simulink model "GVCU_HIL"  (R2026a)
settings: Solver=ode3  StartTime=0  StopTime=2474  FixedStep=0.0002
model workspace (MAT data in the model file):
  CANoelibParameters : object (value not decoded)
values from neighbouring files (symbols this model uses):
  acc_pedal_data = pedal_data.accelerator_pedal_position_t0    [Vehicle_Simulink_init.m]
  acc_pedal_time = pedal_data.t0    [Vehicle_Simulink_init.m]
  brk_pedal_data = brake_pedal_data.shared_brakes_drvrBrkPedlPerc_t0    [Vehicle_Simulink_init.m]
  brk_pedal_time = brake_pedal_data.t0    [Vehicle_Simulink_init.m]
  cycle_len = zeros(1, num_cycles)    [Vehicle_Simulink_init.m]
  cycle_speed_matrix = zeros(max_cycle_len, num_cycles)    [Vehicle_Simulink_init.m]
  cycle_time_matrix = zeros(max_cycle_len, num_cycles)    [Vehicle_Simulink_init.m]
  veh_speed_data = speed_data.shared_dynamicsVso_vehVelLgt_t0    [Vehicle_Simulink_init.m]
  veh_speed_time = speed_data.t0    [Vehicle_Simulink_init.m]
undefined symbols (not defined in the file or in its folder): Active, AuxActive, bat, environment, FL_prs_voltage, FR_prs_voltage, pos, RL_prs_voltage, RR_prs_voltage, tir, veh, VGetRawValueFlag, Voltage, VT2816_1_Ch1, VT2816_1_Ch2, VT2816_1_Ch3, VT2816_1_Ch4, VT2816_3_Ch13, VT2816_3_Ch14, VT7101_1_Out2, VT7820_2_Channel1, VT7820_2_Channel2, VT7820_2_Channel3, VT7820_2_Channel4, VTS
libraries: canoelib x144, autolibsharedcoupling x21, autolibcoupling x9, autolibshared x5, simulink_extras x4, simulink x4, slpidlib x3, autolibshareddiff x3, autolibutils x1, autolibdatasheetbattery x1, autolibmappedmotor x1, sl_discontinuities x1
(part 2 of 9)

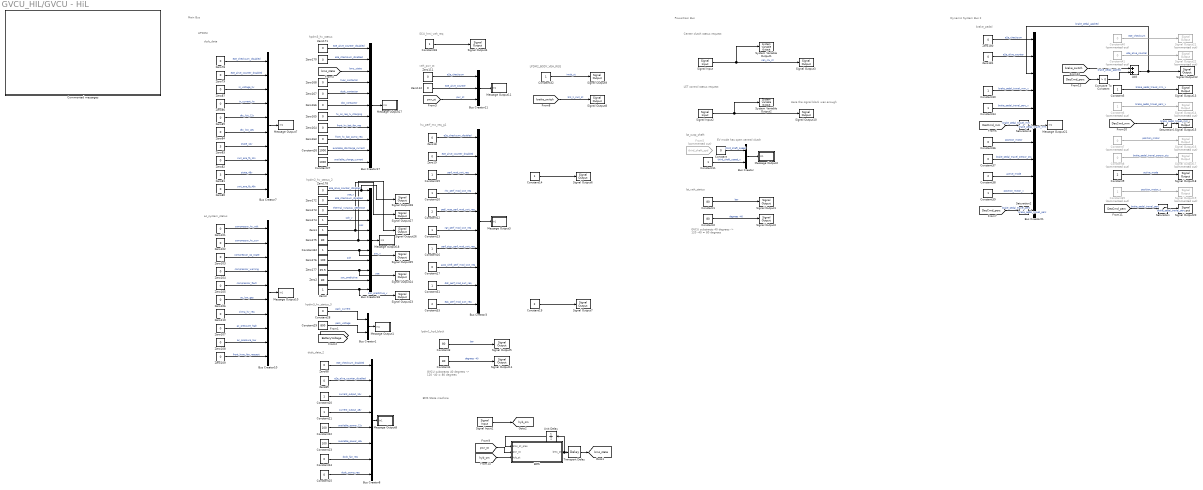
== system GVCU_HIL/GVCU - HiL ==
  note: EV mode has open central clutch
  note: GVCU substracts 40 degrees
      | -> 120 -40 =  80 degrees
  note: hu_perf_mo_req_g1
  note: HPDM3
  note: hpdm2_hv_status_2
  note: dcdc_data
  note: hpdm3_hv_status_3
  note: dcdc_data_2
  note: Here the signal block was enough
  note: ac_system_status
  note: LPDM2_BODY_VEH_REQ
  note: brake_pedal
  note: veh_pwr_st
  note: hpdm3_hv_status
  note: lst_outp_shaft
  note: Powertrain Bus
  note: Center clutch status request
  note: SCU_hmi_veh_req
  note: LST control status request
  note: Main Bus
  note: Dynamic System Bus 2
  note: lst_veh_status
  note: lpdm1_hyd_block
  note: GVCU substracts 40 degrees
      | -> 120 -40 =  80 degrees
  note: BMS State machine
  Add : Sum
  BMS : MATLAB Function  TreatAsAtomicUnit=on
  Bus Creator : BusCreator  Inputs=2
  Bus Creator1 : BusCreator  Inputs=2
  Bus Creator10 : BusCreator  Inputs=10
  Bus Creator11 : BusCreator  Inputs=3
  Bus Creator17 : BusCreator  Inputs=11
  Bus Creator18 : BusCreator  Inputs=11
  Bus Creator21 : BusCreator  Inputs=11
  Bus Creator3 : BusCreator  Inputs=10
  Bus Creator7 : BusCreator  Inputs=10
  Bus Creator8 : BusCreator  Inputs=8
  Commented messages : Subsystem
  Compare To Constant : simulink/Logic and Bit Operations/Compare To Constant  relop=>  const=0  OutDataTypeStr=boolean
  Constant{,17,24..25,28,36..37} (7 alike) : Constant  Value=0
  Constant{1..4} (4 alike) : Constant  Value=80
  Constant{5,10..11,13..16,18,20..21,30..32,34,39,42} (16 alike) : Constant
  Constant{9,12,19,33,38} (5 alike) : Constant  Value=2
  Constant22 : Constant  Value=100
  Constant23 : Constant  Value=100
  Constant26 : Constant  Value=1000
  Constant27 : Constant  Value=1000
  Constant29 : Constant  Value=800
  Constant35 : Constant  Commented=on
  Constant{7..8,40..41} (4 alike) : Constant  Commented=on  Value=0
  Constant6 : Constant  Commented=on
  From5 : From  Commented=on  GotoTag=third_shaft_spd
  Message Output1 : Subsystem  AncestorBlock=canoelib/CANoe I//O/Message Output  mask(Signal Output Module){dbName=main_bus, nodeName=HPDM3, msgName=hpdm3_hv_status_3, inputType=Bus Signal, rawValue=Default}
      mask prompts: dbName "Database name"; nodeName "Node name"; msgName "Message name"; inputType "Input type"; rawValue "Raw value"
      mask help: Output module for all signals of a databasemessage provided by the CANoe interaction layer. Double click the block for configuration.
      settings: AttributesFormatString=%<msgName>  CopyFcn=set_param(gcb, 'AttributesFormatString', '%<msgName>');  OpenFcn=MessageOutputBlock
      mask Help: For detailed information please refer to the CANoe online help 'MATLAB Integration Package » CANoe I/O Library'.
      mask TypeOptions inputType: Vector | Bus Signal
      mask TypeOptions rawValue: Default | Physical value | Raw value
      mask Display:
      | image(imread('MatlabBlock.png'))
      | disp('CANoe')
  Message Output10 : Subsystem  AncestorBlock=canoelib/CANoe I//O/Message Output  mask(Signal Output Module){dbName=main_bus, nodeName=LPDM1, msgName=ac_system_status, inputType=Bus Signal, rawValue=Default}
      mask prompts: dbName "Database name"; nodeName "Node name"; msgName "Message name"; inputType "Input type"; rawValue "Raw value"
      mask help: Output module for all signals of a databasemessage provided by the CANoe interaction layer. Double click the block for configuration.
      settings: AttributesFormatString=%<msgName>  CopyFcn=set_param(gcb, 'AttributesFormatString', '%<msgName>');  OpenFcn=MessageOutputBlock
      mask Help: For detailed information please refer to the CANoe online help 'MATLAB Integration Package » CANoe I/O Library'.
      mask TypeOptions inputType: Vector | Bus Signal
      mask TypeOptions rawValue: Default | Physical value | Raw value
      mask Display:
      | image(imread('MatlabBlock.png'))
      | disp('CANoe')
  Message Output11 : Subsystem  AncestorBlock=canoelib/CANoe I//O/Message Output  mask(Signal Output Module){dbName=main_bus, nodeName=SCU, msgName=veh_pwr_st, inputType=Bus Signal, rawValue=Default}
      mask prompts: dbName "Database name"; nodeName "Node name"; msgName "Message name"; inputType "Input type"; rawValue "Raw value"
      mask help: Output module for all signals of a databasemessage provided by the CANoe interaction layer. Double click the block for configuration.
      settings: AttributesFormatString=veh_pwr_st  CopyFcn=set_param(gcb, 'AttributesFormatString', '%<msgName>');  OpenFcn=MessageOutputBlock
      mask Help: For detailed information please refer to the CANoe online help 'MATLAB Integration Package » CANoe I/O Library'.
      mask TypeOptions inputType: Vector | Bus Signal
      mask TypeOptions rawValue: Default | Physical value | Raw value
      mask Display:
      | image(imread('MatlabBlock.png'))
      | disp('CANoe')
  Message Output17 : Subsystem  AncestorBlock=canoelib/CANoe I//O/Message Output  mask(Signal Output Module){dbName=main_bus, nodeName=HPDM3, msgName=hpdm3_hv_status, inputType=Bus Signal, rawValue=Default}
      mask prompts: dbName "Database name"; nodeName "Node name"; msgName "Message name"; inputType "Input type"; rawValue "Raw value"
      mask help: Output module for all signals of a databasemessage provided by the CANoe interaction layer. Double click the block for configuration.
      settings: AttributesFormatString=%<msgName>  CopyFcn=set_param(gcb, 'AttributesFormatString', '%<msgName>');  OpenFcn=MessageOutputBlock
      mask Help: For detailed information please refer to the CANoe online help 'MATLAB Integration Package » CANoe I/O Library'.
      mask TypeOptions inputType: Vector | Bus Signal
      mask TypeOptions rawValue: Default | Physical value | Raw value
      mask Display:
      | image(imread('MatlabBlock.png'))
      | disp('CANoe')
  Message Output18 : Subsystem  AncestorBlock=canoelib/CANoe I//O/Message Output  mask(Signal Output Module){dbName=main_bus, nodeName=HPDM3, msgName=hpdm3_hv_status_2, inputType=Bus Signal, rawValue=Default}
      mask prompts: dbName "Database name"; nodeName "Node name"; msgName "Message name"; inputType "Input type"; rawValue "Raw value"
      mask help: Output module for all signals of a databasemessage provided by the CANoe interaction layer. Double click the block for configuration.
      settings: AttributesFormatString=hpdm3_hv_status_2  CopyFcn=set_param(gcb, 'AttributesFormatString', '%<msgName>');  OpenFcn=MessageOutputBlock
      mask Help: For detailed information please refer to the CANoe online help 'MATLAB Integration Package » CANoe I/O Library'.
      mask TypeOptions inputType: Vector | Bus Signal
      mask TypeOptions rawValue: Default | Physical value | Raw value
      mask Display:
      | image(imread('MatlabBlock.png'))
      | disp('CANoe')
  Message Output2 : Subsystem  AncestorBlock=canoelib/CANoe I//O/Message Output  mask(Signal Output Module){dbName=powertrain_bus, nodeName=LST, msgName=lst_outp_shaft, inputType=Bus Signal, rawValue=Default}
      mask prompts: dbName "Database name"; nodeName "Node name"; msgName "Message name"; inputType "Input type"; rawValue "Raw value"
      mask help: Output module for all signals of a databasemessage provided by the CANoe interaction layer. Double click the block for configuration.
      settings: AttributesFormatString=%<msgName>  CopyFcn=set_param(gcb, 'AttributesFormatString', '%<msgName>');  OpenFcn=MessageOutputBlock
      mask Help: For detailed information please refer to the CANoe online help 'MATLAB Integration Package » CANoe I/O Library'.
      mask TypeOptions inputType: Vector | Bus Signal
      mask TypeOptions rawValue: Default | Physical value | Raw value
      mask Display:
      | image(imread('MatlabBlock.png'))
      | disp('CANoe')
  Message Output21 : Subsystem  AncestorBlock=canoelib/CANoe I//O/Message Output  mask(Signal Output Module){dbName=dynamic_systems2_bus, nodeName=IEB, msgName=brake_pedal, inputType=Bus Signal, rawValue=Default}
      mask prompts: dbName "Database name"; nodeName "Node name"; msgName "Message name"; inputType "Input type"; rawValue "Raw value"
      mask help: Output module for all signals of a databasemessage provided by the CANoe interaction layer. Double click the block for configuration.
      settings: AttributesFormatString=brake_pedal  CopyFcn=set_param(gcb, 'AttributesFormatString', '%<msgName>');  OpenFcn=MessageOutputBlock
      mask Help: For detailed information please refer to the CANoe online help 'MATLAB Integration Package » CANoe I/O Library'.
      mask TypeOptions inputType: Vector | Bus Signal
      mask TypeOptions rawValue: Default | Physical value | Raw value
      mask Display:
      | image(imread('MatlabBlock.png'))
      | disp('CANoe')
  Message Output3 : Subsystem  AncestorBlock=canoelib/CANoe I//O/Message Output  mask(Signal Output Module){dbName=main_bus, nodeName=SCU, msgName=hu_perf_mod_req_g1, inputType=Bus Signal, rawValue=Default}
      mask prompts: dbName "Database name"; nodeName "Node name"; msgName "Message name"; inputType "Input type"; rawValue "Raw value"
      mask help: Output module for all signals of a databasemessage provided by the CANoe interaction layer. Double click the block for configuration.
      settings: AttributesFormatString=%<msgName>  CopyFcn=set_param(gcb, 'AttributesFormatString', '%<msgName>');  OpenFcn=MessageOutputBlock
      mask Help: For detailed information please refer to the CANoe online help 'MATLAB Integration Package » CANoe I/O Library'.
      mask TypeOptions inputType: Vector | Bus Signal
      mask TypeOptions rawValue: Default | Physical value | Raw value
      mask Display:
      | image(imread('MatlabBlock.png'))
      | disp('CANoe')
  Message Output7 : Subsystem  AncestorBlock=canoelib/CANoe I//O/Message Output  mask(Signal Output Module){dbName=main_bus, nodeName=HPDM3, msgName=dcdc_data, inputType=Bus Signal, rawValue=Default}
      mask prompts: dbName "Database name"; nodeName "Node name"; msgName "Message name"; inputType "Input type"; rawValue "Raw value"
      mask help: Output module for all signals of a databasemessage provided by the CANoe interaction layer. Double click the block for configuration.
      settings: AttributesFormatString=%<msgName>  CopyFcn=set_param(gcb, 'AttributesFormatString', '%<msgName>');  OpenFcn=MessageOutputBlock
      mask Help: For detailed information please refer to the CANoe online help 'MATLAB Integration Package » CANoe I/O Library'.
      mask TypeOptions inputType: Vector | Bus Signal
      mask TypeOptions rawValue: Default | Physical value | Raw value
      mask Display:
      | image(imread('MatlabBlock.png'))
      | disp('CANoe')
  Message Output8 : Subsystem  AncestorBlock=canoelib/CANoe I//O/Message Output  mask(Signal Output Module){dbName=main_bus, nodeName=HPDM3, msgName=dcdc_data_2, inputType=Bus Signal, rawValue=Default}
      mask prompts: dbName "Database name"; nodeName "Node name"; msgName "Message name"; inputType "Input type"; rawValue "Raw value"
      mask help: Output module for all signals of a databasemessage provided by the CANoe interaction layer. Double click the block for configuration.
      settings: AttributesFormatString=%<msgName>  CopyFcn=set_param(gcb, 'AttributesFormatString', '%<msgName>');  OpenFcn=MessageOutputBlock
      mask Help: For detailed information please refer to the CANoe online help 'MATLAB Integration Package » CANoe I/O Library'.
      mask TypeOptions inputType: Vector | Bus Signal
      mask TypeOptions rawValue: Default | Physical value | Raw value
      mask Display:
      | image(imread('MatlabBlock.png'))
      | disp('CANoe')
  Saturation : Saturate  UpperLimit=100  LowerLimit=0
  Saturation1 : Saturate  UpperLimit=25.5  LowerLimit=0
  Saturation2 : Saturate  UpperLimit=100  LowerLimit=0
  Saturation3 : Saturate  UpperLimit=25.5  LowerLimit=0
  Signal Input : canoelib/CANoe I//O/Signal Input  dbName=powertrain_bus  nodeName=GVCU  msgName=gvcu_lst_req  sigName=cen_clu_st_req  editSampleTime=0  rawValue=Default  dataType=Default  dataTypeDB=uint8  hasEncoding=off
      settings: AttributesFormatString=%<sigName>  SourceProductName=Vector CANoe
  Signal Input1 : canoelib/CANoe I//O/Signal Input  dbName=main_bus  nodeName=GVCU  msgName=gvcu_hv_control  sigName=hyb_st_mac_state  editSampleTime=0  rawValue=Default  dataType=Default  dataTypeDB=uint8  hasEncoding=off
      settings: AttributesFormatString=%<sigName>  SourceProductName=Vector CANoe
  Signal Input2 : canoelib/CANoe I//O/Signal Input  dbName=powertrain_bus  nodeName=GVCU  msgName=gvcu_lst_req  sigName=lst_ctrl_st_req  editSampleTime=0  rawValue=Default  dataType=Default  dataTypeDB=uint8  hasEncoding=off
      settings: AttributesFormatString=%<sigName>  SourceProductName=Vector CANoe
  Signal Output1 : canoelib/CANoe I//O/Signal Output  dbName=powertrain_bus  nodeName=LST  msgName=lst_veh_status  sigName=re_hi_p_sys_p  rawValue=Default  dataType=Default  dataTypeDB=uint8  hasEncoding=off
      settings: AttributesFormatString=%<sigName>  SourceProductName=Vector CANoe
  Signal Output10 : canoelib/CANoe I//O/Signal Output  dbName=powertrain_bus  nodeName=LST  msgName=lst_tq_sts_1  sigName=lst_ctrl_st  rawValue=Default  dataType=Default  dataTypeDB=uint8  hasEncoding=off
      settings: AttributesFormatString=%<sigName>  SourceProductName=Vector CANoe
  Signal Output11 : canoelib/CANoe I//O/Signal Output  dbName=main_bus  nodeName=LPDM1  msgName=lpdm1_hyd_block  sigName=autoskin_oil_temperature  rawValue=Default  dataType=Default  dataTypeDB=uint8  hasEncoding=on
      settings: AttributesFormatString=%<sigName>  SourceProductName=Vector CANoe
  Signal Output12 : canoelib/CANoe I//O/Signal Output  dbName=dynamic_systems2_bus  nodeName=IEB  msgName=brake_pedal  sigName=brake_pedal_applied  rawValue=Default  dataType=Default  dataTypeDB=uint8  hasEncoding=off
      settings: AttributesFormatString=%<sigName>  SourceProductName=Vector CANoe
  Signal Output13 : canoelib/CANoe I//O/Signal Output  dbName=dynamic_systems2_bus  nodeName=IEB  msgName=brake_pedal  sigName=brake_pedal_travel_mm_v  rawValue=Default  dataType=Default  dataTypeDB=boolean  hasEncoding=off
      settings: AttributesFormatString=%<sigName>  SourceProductName=Vector CANoe
  Signal Output14 : canoelib/CANoe I//O/Signal Output  Commented=on  dbName=dynamic_systems2_bus  nodeName=IEB  msgName=brake_pedal  sigName=brake_pedal_travel_perc_v  rawValue=Default  dataType=Default  dataTypeDB=boolean  hasEncoding=off
      settings: AttributesFormatString=%<sigName>  SourceProductName=Vector CANoe
  Signal Output15 : canoelib/CANoe I//O/Signal Output  dbName=dynamic_systems2_bus  nodeName=IEB  msgName=brake_pedal  sigName=brake_pedal_travel_mm  rawValue=Default  dataType=Default  dataTypeDB=uint8  hasEncoding=on
      settings: AttributesFormatString=%<sigName>  SourceProductName=Vector CANoe
  Signal Output16 : canoelib/CANoe I//O/Signal Output  Commented=on  dbName=dynamic_systems2_bus  nodeName=IEB  msgName=brake_pedal  sigName=brake_pedal_travel_perc_v  rawValue=Default  dataType=Default  dataTypeDB=boolean  hasEncoding=off
      settings: AttributesFormatString=%<sigName>  SourceProductName=Vector CANoe
  Signal Output17 : canoelib/CANoe I//O/Signal Output  Commented=on  dbName=dynamic_systems2_bus  nodeName=IEB  msgName=brake_pedal  sigName=brake_pedal_travel_sensor_sts  rawValue=Default  dataType=Default  dataTypeDB=uint8  hasEncoding=off
      settings: AttributesFormatString=%<sigName>  SourceProductName=Vector CANoe
  Signal Output18 : canoelib/CANoe I//O/Signal Output  dbName=dynamic_systems2_bus  nodeName=IEB  msgName=brake_pedal  sigName=active_mode  rawValue=Default  dataType=Default  dataTypeDB=uint8  hasEncoding=off
      settings: AttributesFormatString=%<sigName>  SourceProductName=Vector CANoe
  Signal Output19 : canoelib/CANoe I//O/Signal Output  Commented=on  dbName=dynamic_systems2_bus  nodeName=IEB  msgName=brake_pedal  sigName=position_motor_v  rawValue=Default  dataType=Default  dataTypeDB=boolean  hasEncoding=off
      settings: AttributesFormatString=%<sigName>  SourceProductName=Vector CANoe
  Signal Output2 : canoelib/CANoe I//O/Signal Output  dbName=powertrain_bus  nodeName=LST  msgName=lst_veh_status  sigName=re_hi_p_sys_t  rawValue=Default  dataType=Default  dataTypeDB=uint8  hasEncoding=on
      settings: AttributesFormatString=%<sigName>  SourceProductName=Vector CANoe
  Signal Output20 : canoelib/CANoe I//O/Signal Output  dbName=dynamic_systems2_bus  nodeName=IEB  msgName=brake_pedal  sigName=brake_pedal_travel_perc  rawValue=Default  dataType=Default  dataTypeDB=uint16  hasEncoding=on
      settings: AttributesFormatString=%<sigName>  SourceProductName=Vector CANoe
  Signal Output21 : canoelib/CANoe I//O/Signal Output  Commented=on  dbName=dynamic_systems2_bus  nodeName=IEB  msgName=brake_pedal  sigName=e2e_checksum  rawValue=Default  dataType=Default  dataTypeDB=uint8  hasEncoding=off
      settings: AttributesFormatString=%<sigName>  SourceProductName=Vector CANoe
  Signal Output22 : canoelib/CANoe I//O/Signal Output  Commented=on  dbName=dynamic_systems2_bus  nodeName=IEB  msgName=brake_pedal  sigName=e2e_alive_counter  rawValue=Default  dataType=Default  dataTypeDB=uint8  hasEncoding=off
      settings: AttributesFormatString=%<sigName>  SourceProductName=Vector CANoe
  Signal Output23 : canoelib/CANoe I//O/Signal Output  dbName=main_bus  nodeName=HPDM3  msgName=hpdm3_hv_status_2  sigName=soc_predictive_v  rawValue=Default  dataType=Default  dataTypeDB=boolean  hasEncoding=off
      settings: AttributesFormatString=%<sigName>  SourceProductName=Vector CANoe
  Signal Output24 : canoelib/CANoe I//O/Signal Output  dbName=main_bus  nodeName=HPDM3  msgName=hpdm3_hv_status_2  sigName=soe  rawValue=Default  dataType=Default  dataTypeDB=uint8  hasEncoding=on
      settings: AttributesFormatString=%<sigName>  SourceProductName=Vector CANoe
  Signal Output25 : canoelib/CANoe I//O/Signal Output  dbName=main_bus  nodeName=HPDM3  msgName=hpdm3_hv_status_2  sigName=soc_v  rawValue=Default  dataType=Default  dataTypeDB=boolean  hasEncoding=off
      settings: AttributesFormatString=%<sigName>  SourceProductName=Vector CANoe
  Signal Output26 : canoelib/CANoe I//O/Signal Output  dbName=main_bus  nodeName=HPDM3  msgName=hpdm3_hv_status_2  sigName=soc  rawValue=Default  dataType=Default  dataTypeDB=uint16  hasEncoding=on
      settings: AttributesFormatString=%<sigName>  SourceProductName=Vector CANoe
  Signal Output27 : canoelib/CANoe I//O/Signal Output  dbName=main_bus  nodeName=HPDM3  msgName=hpdm3_hv_status_2  sigName=soe_v  rawValue=Default  dataType=Default  dataTypeDB=boolean  hasEncoding=off
      settings: AttributesFormatString=%<sigName>  SourceProductName=Vector CANoe
  Signal Output28 : canoelib/CANoe I//O/Signal Output  dbName=main_bus  nodeName=HPDM3  msgName=hpdm3_hv_status_2  sigName=e2e_alive_counter_disabled  rawValue=Default  dataType=Default  dataTypeDB=uint8  hasEncoding=off
      settings: AttributesFormatString=%<sigName>  SourceProductName=Vector CANoe
  Signal Output3 : canoelib/CANoe I//O/Signal Output  dbName=powertrain_bus  nodeName=LST  msgName=lst_tq_sts_2  sigName=cen_clu_st  rawValue=Default  dataType=Default  dataTypeDB=uint8  hasEncoding=off
      settings: AttributesFormatString=%<sigName>  SourceProductName=Vector CANoe
  Signal Output4 : canoelib/CANoe I//O/Signal Output  dbName=main_bus  nodeName=SCU  msgName=scu_hmi_veh_req  sigName=suppg_mod_req  rawValue=Default  dataType=Default  dataTypeDB=uint8  hasEncoding=off
      settings: AttributesFormatString=%<sigName>  SourceProductName=Vector CANoe
  Signal Output5 : canoelib/CANoe I//O/Signal Output  dbName=main_bus  nodeName=LPDM1  msgName=lpdm1_hyd_block  sigName=autoskin_oil_pressure  rawValue=Default  dataType=Default  dataTypeDB=uint16  hasEncoding=on
      settings: AttributesFormatString=%<sigName>  SourceProductName=Vector CANoe
  Signal Output6 : canoelib/CANoe I//O/Signal Output  dbName=main_bus  nodeName=SCU  msgName=hu_perf_mod_req_g1  sigName=perf_mod_swt_req  rawValue=Default  dataType=Default  dataTypeDB=uint8  hasEncoding=off
      settings: AttributesFormatString=%<sigName>  SourceProductName=Vector CANoe
  Signal Output7 : canoelib/CANoe I//O/Signal Output  dbName=main_bus  nodeName=SCU  msgName=hu_perf_mod_req_g1  sigName=eps_perf_mod_swt_req  rawValue=Default  dataType=Default  dataTypeDB=uint8  hasEncoding=off
      settings: AttributesFormatString=%<sigName>  SourceProductName=Vector CANoe
  Signal Output8 : canoelib/CANoe I//O/Signal Output  dbName=main_bus  nodeName=LPDM2  msgName=lpdm2_body_veh_req  sigName=brk_li_swt_st  rawValue=Default  dataType=Default  dataTypeDB=uint8  hasEncoding=off
      settings: AttributesFormatString=%<sigName>  SourceProductName=Vector CANoe
  Signal Output9 : canoelib/CANoe I//O/Signal Output  dbName=main_bus  nodeName=LPDM2  msgName=lpdm2_body_veh_req  sigName=imob_st  rawValue=Default  dataType=Default  dataTypeDB=uint8  hasEncoding=off
      settings: AttributesFormatString=%<sigName>  SourceProductName=Vector CANoe
  System Variable Output1 : canoelib/CANoe I//O/System Variable Output  nsName=Checker_Simulink  sysVarName=cen_clu_st  arrayIndex=-1  rawValue=Default  dataType=Default  dataTypeDB=int32  hasEncoding=off  dataTypeCANoe=Get from CANoe
      settings: AttributesFormatString=%<nsName>::%<sysVarName>  SourceProductName=Vector CANoe
  System Variable Output2 : canoelib/CANoe I//O/System Variable Output  nsName=Checker_Simulink  sysVarName=lst_ctrl_st  arrayIndex=-1  rawValue=Default  dataType=Default  dataTypeDB=int32  hasEncoding=off  dataTypeCANoe=Get from CANoe
      settings: AttributesFormatString=%<nsName>::%<sysVarName>  SourceProductName=Vector CANoe
  Transport Delay : TransportDelay
  Unit Delay : UnitDelay  SampleTime=-1
  Zero1 : Constant  OutDataTypeStr=Inherit: Inherit via back propagation
  Zero{18..19,78..80,82,84..89,101..112,163..168,170..173,178,180..181} (37 alike) : Constant  Value=0  OutDataTypeStr=Inherit: Inherit via back propagation
  Zero174 : Constant  OutDataTypeStr=Inherit: Inherit via back propagation
  Zero175 : Constant  Value=80  OutDataTypeStr=Inherit: Inherit via back propagation
  Zero176 : Constant  Value=100  OutDataTypeStr=Inherit: Inherit via back propagation
  Zero177 : Constant  Value=25.5  OutDataTypeStr=Inherit: Inherit via back propagation
  Zero2 : Constant  Value=80  OutDataTypeStr=Inherit: Inherit via back propagation
  Zero3 : Constant  OutDataTypeStr=Inherit: Inherit via back propagation
  Zero81 : Constant  Value=3  OutDataTypeStr=Inherit: Inherit via back propagation
  Zero83 : Constant  Value=3  OutDataTypeStr=Inherit: Inherit via back propagation
  tag scope: bms_state=global, hyb_sm=global
  wires:
  Zero165/1 -> Bus Creator17/7  "hv_on_req_lv_charging"
  Zero104/1 -> Bus Creator10/4  "compressor_warning"
  Constant38/1 -> Bus Creator21/9  "active_mode"
  Zero103/1 -> Bus Creator10/3  "compressor_op_state"
  Zero109/1 -> Bus Creator10/10  "front_hvac_fan_request"
  Constant34/1 -> Bus Creator21/5  "brake_pedal_travel_perc_v"
  Constant33/1 -> Bus Creator3/10  "eps_perf_mod_swt_req"
  Zero79/1 -> Bus Creator7/2  "e2e_alive_counter_disabled"
  Constant30/1 -> Bus Creator21/4  "brake_pedal_travel_mm_v"
  Zero173/1 -> Bus Creator18/3  "thermal_runaway_detection"
  Constant16/1 -> Bus Creator3/7  "perf_stgy_perf_mod_swt_req"
  Zero180/1 -> Bus Creator21/1  "e2e_checksum"
  [bms_state] -> Bus Creator17/3  "bms_state"
  Zero164/1 -> Bus Creator17/8  "front_hv_bat_fan_req"
  Constant22/1 -> Bus Creator8/5  "available_power_12v"
  Constant36/1 -> Bus Creator21/7  "position_motor"
  Constant24/1 -> Bus Creator8/7  "dcdc_fan_req"
  Constant31/1 -> Bus Creator3/9  "ddc_perf_mod_swt_req"
  Constant39/1 -> Bus Creator21/10  "position_motor_v"
  Constant15/1 -> Bus Creator3/3  "perf_mod_swt_req"
  Bus Creator18/1 -> Message Output18/1(In1)
  Zero111/1 -> Bus Creator11/1  "e2e_checksum"
  Zero86/1 -> Bus Creator7/4  "in_current_hv"
  Constant37/1 -> Bus Creator21/8  "brake_pedal_travel_sensor_sts"
  Zero81/1 -> Bus Creator7/9  "state_48v"
  Zero83/1 -> Bus Creator7/7  "state_12v"
  Constant21/1 -> Bus Creator8/4  "current_output_48v"
  Zero177/1 -> Signal Output24/1, Bus Creator18/9  "soe"
  Zero89/1 -> Bus Creator8/2  "e2e_alive_counter_disabled"
  Signal Input/1 -> Signal Output3/1, System Variable Output1/1  "cen_clu_st"
  Zero88/1 -> Bus Creator8/1  "e2e_checksum_disabled"
  Constant14/1 -> Signal Output6/1
  Bus Creator3/1 -> Message Output3/1(In1)
  Zero176/1 -> Bus Creator18/8  "soh"
  Zero80/1 -> Bus Creator7/10  "swt_ena_fb_48v"
  Zero178/1 -> Signal Output28/1, Bus Creator18/1  "e2e_alive_counter_disabled"
  Zero101/1 -> Bus Creator10/1  "compressor_hv_volt"
  Zero168/1 -> Bus Creator17/4  "hvac_contactor"
  Zero175/1 -> Signal Output26/1, Bus Creator18/6  "soc"
  Bus Creator1/1 -> Message Output1/1(In1)
  Add/1 -> Bus Creator21/3, Signal Output12/1  "brake_pedal_applied"
  Zero18/1 -> Bus Creator3/1  "e2e_checksum_disabled"
  Constant19/1 -> Signal Output7/1
  Zero181/1 -> Bus Creator21/2  "e2e_alive_counter"
  Zero105/1 -> Bus Creator10/5  "compressor_fault"
  Bus Creator7/1 -> Message Output7/1(In1)
  Zero87/1 -> Bus Creator7/3  "in_voltage_hv"
  Constant18/1 -> Signal Output4/1
  Zero82/1 -> Bus Creator7/8  "swt_ena_fb_12v"
  Zero163/1 -> Bus Creator17/9  "front_hv_bat_pump_req"
  Constant27/1 -> Bus Creator17/11  "available_charge_current"
  Zero19/1 -> Bus Creator3/2  "e2e_alive_counter_disabled"
  Bus Creator10/1 -> Message Output10/1(In1)
  Constant26/1 -> Bus Creator17/10  "available_discharge_current"
  Zero174/1 -> Bus Creator18/4  "soh_v"
  Bus Creator11/1 -> Message Output11/1(In1)
  [DecCmd_mm] -> Saturation3/1  "brake_pedal_travel_mm"
  [DecCmd_perc] -> Saturation2/1  "brake_pedal_travel_perc"
  Bus Creator8/1 -> Message Output8/1(In1)
  Constant11/1 -> Bus Creator/2  "third_shaft_speed_v"
  Zero112/1 -> Bus Creator11/2  "e2e_alive_counter"
  Constant29/1 -> Bus Creator1/2  "pack_voltage"
  Constant12/1 -> Bus Creator3/5  "pedl_map_perf_mod_swt_req"
  Zero107/1 -> Bus Creator10/8  "ac_pressure_high"
  Zero170/1 -> Bus Creator17/2  "e2e_checksum_disabled"
  Zero171/1 -> Bus Creator17/1  "e2e_alive_counter_disabled"
  Constant25/1 -> Bus Creator8/8  "dcdc_pump_req"
  Zero85/1 -> Bus Creator7/5  "dtc_list_12v"
  Constant23/1 -> Bus Creator8/6  "available_power_48v"
  Constant13/1 -> Bus Creator3/6  "rgn_perf_mod_swt_req"
  Zero102/1 -> Bus Creator10/2  "compressor_hv_curr"
  Constant/1 -> Bus Creator/1  "third_shaft_speed"
  Constant32/1 -> Signal Output9/1  "imob_st"
  Constant17/1 -> Bus Creator3/8  "auto_shift_perf_mod_swt_req"
  [pwr_st] -> Bus Creator11/3  "pwr_st"
  Zero167/1 -> Bus Creator17/5  "dcdc_contactor"
  Zero108/1 -> Bus Creator10/9  "ac_pressure_low"
  Zero110/1 -> Bus Creator10/7  "clima_hv_req"
  Zero172/1 -> Bus Creator18/2  "e2e_checksum_disabled"
  Zero84/1 -> Bus Creator7/6  "dtc_list_48v"
  Constant10/1 -> Bus Creator3/4  "rhc_perf_mod_swt_req"
  Zero78/1 -> Bus Creator7/1  "e2e_checksum_disabled"
  Zero166/1 -> Bus Creator17/6  "obc_contactor"
  Bus Creator/1 -> Message Output2/1(In1)
  Zero106/1 -> Bus Creator10/6  "ac_low_gas"
  Constant20/1 -> Bus Creator8/3  "current_output_12v"
  Constant28/1 -> Bus Creator1/1  "pack_current"
  Bus Creator21/1 -> Message Output21/1(In1)
  [brake_switch] -> Signal Output8/1  "brk_li_swt_st"
  Signal Input2/1 -> System Variable Output2/1, Signal Output10/1
  Bus Creator17/1 -> Message Output17/1(In1)
  Constant1/1 -> Signal Output1/1  "bar"
  Constant2/1 -> Signal Output2/1  "degrees -40"
  Constant3/1 -> Signal Output5/1  "bar"
  Constant4/1 -> Signal Output11/1  "degrees -40"
  [DecCmd_mm] -> Saturation1/1
  Constant35/1 -> Signal Output19/1  "position_motor_v"
  [DecCmd_perc] -> Saturation/1  "brake_pedal_travel_perc"
  Constant6/1 -> Signal Output14/1  "brake_pedal_travel_perc_v"
  Constant8/1 -> Signal Output17/1  "brake_pedal_travel_sensor_sts"
  Constant7/1 -> Signal Output16/1  "position_motor"
  Constant9/1 -> Signal Output18/1  "active_mode"
  Constant5/1 -> Signal Output13/1  "brake_pedal_travel_mm_v"
  Constant40/1 -> Signal Output21/1  "e2e_checksum"
  Constant41/1 -> Signal Output22/1  "e2e_alive_counter"
  Saturation/1 -> Signal Output20/1  "brake_pedal_travel_perc"
  Saturation1/1 -> Signal Output15/1  "brake_pedal_travel_mm"
  Saturation2/1 -> Bus Creator21/11  "brake_pedal_travel_perc"
  Saturation3/1 -> Bus Creator21/6  "brake_pedal_travel_mm"
  [brake_switch] -> Add/1  "brake_pedal_applied"
  Compare To Constant/1 -> Add/2
  [DecCmd_perc] -> Compare To Constant/1
  BMS/1(bms_st) -> Unit Delay/1, Transport Delay/1
  Transport Delay/1 -> [bms_state]
  [hyb_sm] -> BMS/3(hyb_st)
  [pwr_st] -> BMS/2(pwr_st)
  Unit Delay/1 -> BMS/1(bms_st_prev)
  Signal Input1/1 -> [hyb_sm]
  Constant42/1 -> Signal Output25/1, Bus Creator18/7  "soc_v"
  Zero1/1 -> Signal Output27/1, Bus Creator18/5  "soe_v"
  Zero2/1 -> Bus Creator18/10  "soc_predictive"
  Zero3/1 -> Signal Output23/1, Bus Creator18/11  "soc_predictive_v"
